simulink model "simulation_car"  (R2020b)
settings: Solver=VariableStepAuto  StartTime=0.0  StopTime=5  RelTol=1e-3
values from neighbouring files (symbols this model uses):
  InitialPosition = zeros(3,1)    [InitSimulink.m]
  InitialVelocity = zeros(3,1)    [InitSimulink.m]
undefined symbols (not defined in the file or in its folder): param
libraries: aerolibutil x10, sharedtransform x6, vrlib x2
settings Model: Creator=rt-2pm2  LastModifiedBy=rt-2pm2

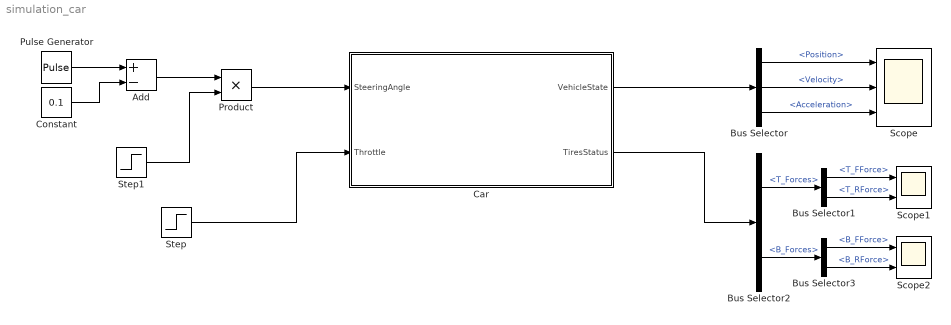
== system simulation_car ==
  Add : Sum  Inputs=+-
  Bus Selector : BusSelector  OutputSignals=StateTranslational.Position,StateTranslational.Velocity,StateTranslational.Acceleration
  Bus Selector1 : BusSelector  OutputSignals=T_FForce,T_RForce
  Bus Selector2 : BusSelector  OutputSignals=T_Forces,B_Forces
  Bus Selector3 : BusSelector  OutputSignals=B_FForce,B_RForce
  Car : Subsystem
  Constant : Constant  Value=0.1
  Product : Product
  Pulse Generator : DiscretePulseGenerator  PulseType=Time based  Amplitude=0.2  Period=10  PulseWidth=5
  Scope : Scope  NumInputPorts=3
  Scope1 : Scope  NumInputPorts=2
  Scope2 : Scope  NumInputPorts=2
  Step : Step  Time=3  Before=3  After=0  SampleTime=0
  Step1 : Step  Time=2  SampleTime=0
  wires:
  Pulse Generator/1 -> Add/1
  Step/1 -> Car/2(Throttle)
  Car/1(VehicleState) -> Bus Selector/1
  Bus Selector/1 -> Scope/1  "<Position>"
  Bus Selector/2 -> Scope/2  "<Velocity>"
  Bus Selector/3 -> Scope/3  "<Acceleration>"
  Car/2(TiresStatus) -> Bus Selector2/1
  Bus Selector1/1 -> Scope1/1  "<T_FForce>"
  Bus Selector1/2 -> Scope1/2  "<T_RForce>"
  Bus Selector2/1 -> Bus Selector1/1  "<T_Forces>"
  Bus Selector3/2 -> Scope2/2  "<B_RForce>"
  Bus Selector3/1 -> Scope2/1  "<B_FForce>"
  Bus Selector2/2 -> Bus Selector3/1  "<B_Forces>"
  Add/1 -> Product/1
  Constant/1 -> Add/2
  Product/1 -> Car/1(SteeringAngle)
  Step1/1 -> Product/2

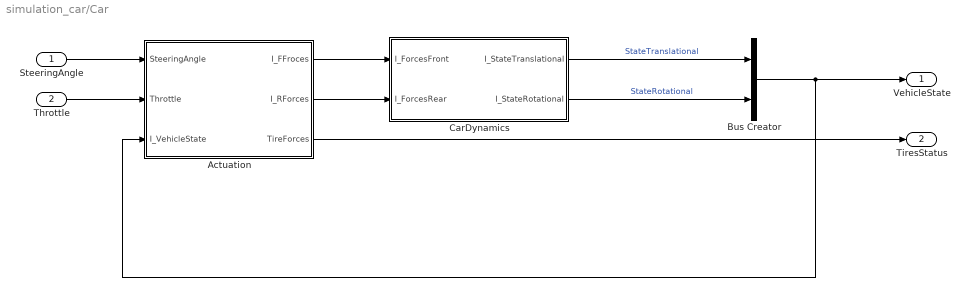
== system simulation_car/Car ==
  SteeringAngle : Inport
  Throttle : Inport  Port=2
  Actuation : Subsystem
  Bus Creator : BusCreator  Inputs=2
  CarDynamics : Subsystem  mask{CarMass=param.m, FrontArmLength=param.a, RearArmLength=param.b, MomentOfInertia=param.Iz}
      mask prompts: CarMass "Car Mass"; FrontArmLength "Front Arm Length"; RearArmLength "Rear Arm Length"; MomentOfInertia "Rotational Inertia"
  VehicleState : Outport
  TiresStatus : Outport  Port=2
  wires:
  CarDynamics/2(I_StateRotational) -> Bus Creator/2  "StateRotational"
  SteeringAngle/1 -> Actuation/1(SteeringAngle)
  CarDynamics/1(I_StateTranslational) -> Bus Creator/1  "StateTranslational"
  Bus Creator/1 -> VehicleState/1, Actuation/3(I_VehicleState)
  Actuation/1(I_FFroces) -> CarDynamics/1(I_ForcesFront)
  Throttle/1 -> Actuation/2(Throttle)
  Actuation/2(I_RForces) -> CarDynamics/2(I_ForcesRear)
  Actuation/3(TireForces) -> TiresStatus/1

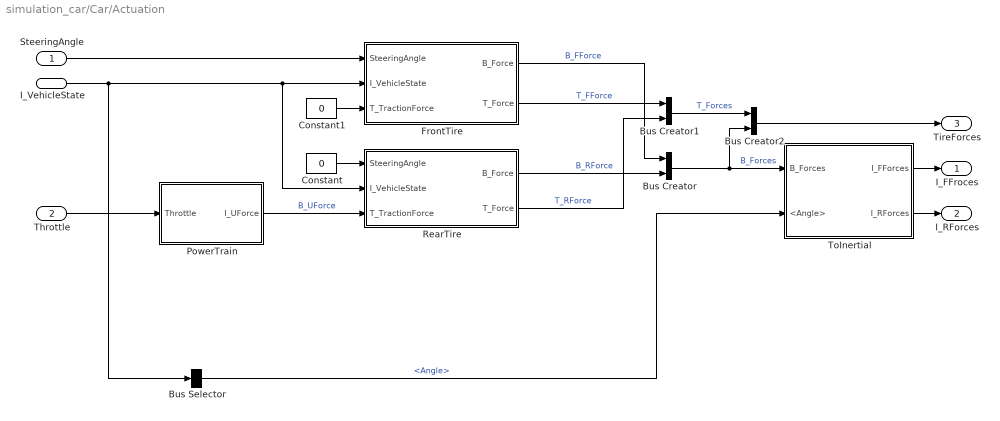
== system simulation_car/Car/Actuation ==
  SteeringAngle : Inport
  Throttle : Inport  Port=2
  I_VehicleState : Inport  Port=3
  Bus Creator : BusCreator  Inputs=2
  Bus Creator1 : BusCreator  Inputs=2
  Bus Creator2 : BusCreator  Inputs=2
  Bus Selector : BusSelector  OutputSignals=StateRotational.Angle
  Constant : Constant  Value=0
  Constant1 : Constant  Value=0
  FrontTire : Subsystem  mask{Arm=[param.a; 0; 0], TireCoeff=param.C_af}
      mask prompts: Arm "Wheel Displacement"; TireCoeff "Tire Coefficient"
      mask Display: image('/home/rt-2pm2/Documents/MATLAB/CIS/lanekeeping_supervision/Simulink/images/tire2.png'); % Use "Edit Image" on toolstrip to change.
  PowerTrain : Subsystem
  RearTire : Subsystem  mask{Arm=[param.a; 0; 0], TireCoeff=param.C_af}
      mask prompts: Arm "Wheel Displacement"; TireCoeff "Tire Coefficient"
      mask Display: image('/home/rt-2pm2/Documents/MATLAB/CIS/lanekeeping_supervision/Simulink/images/tire2.png'); % Use "Edit Image" on toolstrip to change.
  ToInertial : Subsystem
  I_FFroces : Outport
  I_RForces : Outport  Port=2
  TireForces : Outport  Port=3
  wires:
  PowerTrain/1(I_UForce) -> RearTire/3(T_TractionForce)  "B_UForce"
  SteeringAngle/1 -> FrontTire/1(SteeringAngle)
  Throttle/1 -> PowerTrain/1(Throttle)
  I_VehicleState/1 -> Bus Selector/1, RearTire/2(I_VehicleState), FrontTire/2(I_VehicleState)
  Constant/1 -> RearTire/1(SteeringAngle)
  FrontTire/1(B_Force) -> Bus Creator/1  "B_FForce"
  RearTire/1(B_Force) -> Bus Creator/2  "B_RForce"
  Bus Selector/1 -> ToInertial/2(<Angle>)  "<Angle>"
  ToInertial/2(I_RForces) -> I_RForces/1
  ToInertial/1(I_FForces) -> I_FFroces/1
  Constant1/1 -> FrontTire/3(T_TractionForce)
  Bus Creator/1 -> Bus Creator2/2, ToInertial/1(B_Forces)  "B_Forces"
  FrontTire/2(T_Force) -> Bus Creator1/1  "T_FForce"
  RearTire/2(T_Force) -> Bus Creator1/2  "T_RForce"
  Bus Creator1/1 -> Bus Creator2/1  "T_Forces"
  Bus Creator2/1 -> TireForces/1

== system simulation_car/Car/CarDynamics ==
  I_ForcesFront : Inport
  I_ForcesRear : Inport  Port=2
  Subsystem : Subsystem
  Subsystem1 : Subsystem
  I_StateTranslational : Outport
  I_StateRotational : Outport  Port=2
  wires:
  Subsystem/1(StateRotational) -> I_StateRotational/1
  I_ForcesFront/1 -> Subsystem/1(FrontForce), Subsystem1/1(FrontForce)
  I_ForcesRear/1 -> Subsystem/2(RearForce), Subsystem1/2(RearForce)
  Subsystem1/1(StateTranslational) -> I_StateTranslational/1

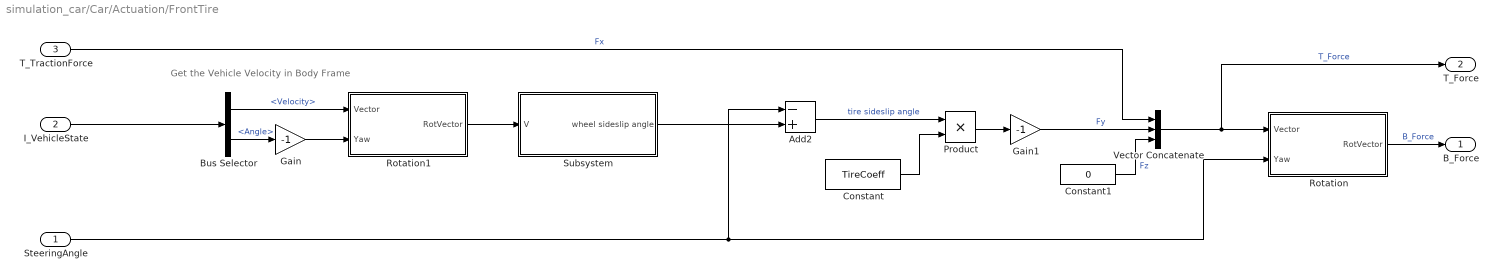
== system simulation_car/Car/Actuation/FrontTire ==
  note: Get the Vehicle Velocity in Body Frame
  SteeringAngle : Inport
  I_VehicleState : Inport  Port=2
  T_TractionForce : Inport  Port=3
  Add2 : Sum  Inputs=-+
  Bus Selector : BusSelector  OutputSignals=StateTranslational.Velocity,StateRotational.Angle
  Constant : Constant  Value=TireCoeff
  Constant1 : Constant  Value=0
  Gain : Gain  Gain=-1
  Gain1 : Gain  Gain=-1
  Product : Product
  Rotation : Subsystem
  Rotation1 : Subsystem
  Subsystem : Subsystem
  Vector Concatenate : Concatenate  NumInputs=3
  B_Force : Outport
  T_Force : Outport  Port=2
  wires:
  Vector Concatenate/1 -> T_Force/1, Rotation/1(Vector)  "T_Force"
  Gain1/1 -> Vector Concatenate/2  "Fy"
  Product/1 -> Gain1/1
  Constant/1 -> Product/2
  Bus Selector/1 -> Rotation1/1(Vector)  "<Velocity>"
  Gain/1 -> Rotation1/2(Yaw)
  Bus Selector/2 -> Gain/1  "<Angle>"
  I_VehicleState/1 -> Bus Selector/1
  Add2/1 -> Product/1  "tire sideslip angle"
  T_TractionForce/1 -> Vector Concatenate/1  "Fx"
  SteeringAngle/1 -> Rotation/2(Yaw), Add2/1
  Rotation/1(RotVector) -> B_Force/1  "B_Force"
  Constant1/1 -> Vector Concatenate/3  "Fz"
  Rotation1/1(RotVector) -> Subsystem/1(V)
  Subsystem/1(wheel sideslip angle) -> Add2/2

== system simulation_car/Car/Actuation/PowerTrain ==
  Throttle : Inport
  Throttle2Force : Gain
  I_UForce : Outport
  wires:
  Throttle/1 -> Throttle2Force/1
  Throttle2Force/1 -> I_UForce/1

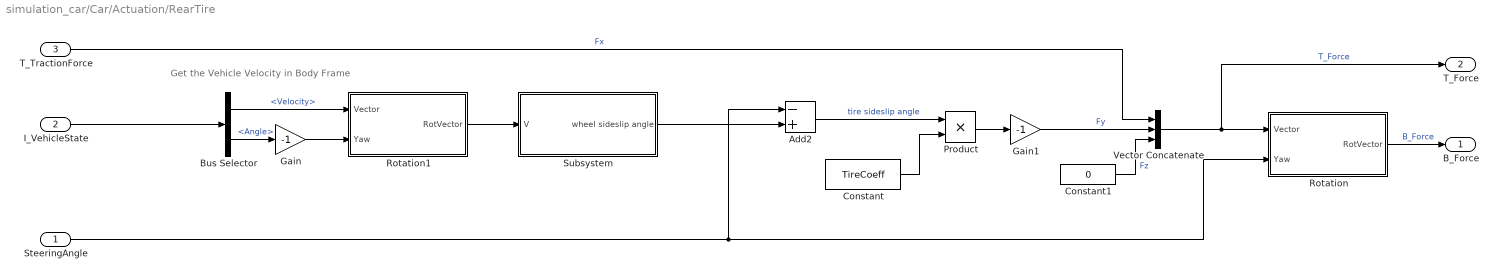
== system simulation_car/Car/Actuation/RearTire ==
  note: Get the Vehicle Velocity in Body Frame
  SteeringAngle : Inport
  I_VehicleState : Inport  Port=2
  T_TractionForce : Inport  Port=3
  Add2 : Sum  Inputs=-+
  Bus Selector : BusSelector  OutputSignals=StateTranslational.Velocity,StateRotational.Angle
  Constant : Constant  Value=TireCoeff
  Constant1 : Constant  Value=0
  Gain : Gain  Gain=-1
  Gain1 : Gain  Gain=-1
  Product : Product
  Rotation : Subsystem
  Rotation1 : Subsystem
  Subsystem : Subsystem
  Vector Concatenate : Concatenate  NumInputs=3
  B_Force : Outport
  T_Force : Outport  Port=2
  wires:
  Subsystem/1(wheel sideslip angle) -> Add2/2
  Rotation1/1(RotVector) -> Subsystem/1(V)
  Constant1/1 -> Vector Concatenate/3  "Fz"
  Rotation/1(RotVector) -> B_Force/1  "B_Force"
  SteeringAngle/1 -> Add2/1, Rotation/2(Yaw)
  T_TractionForce/1 -> Vector Concatenate/1  "Fx"
  Add2/1 -> Product/1  "tire sideslip angle"
  I_VehicleState/1 -> Bus Selector/1
  Bus Selector/2 -> Gain/1  "<Angle>"
  Gain/1 -> Rotation1/2(Yaw)
  Bus Selector/1 -> Rotation1/1(Vector)  "<Velocity>"
  Constant/1 -> Product/2
  Product/1 -> Gain1/1
  Gain1/1 -> Vector Concatenate/2  "Fy"
  Vector Concatenate/1 -> Rotation/1(Vector), T_Force/1  "T_Force"

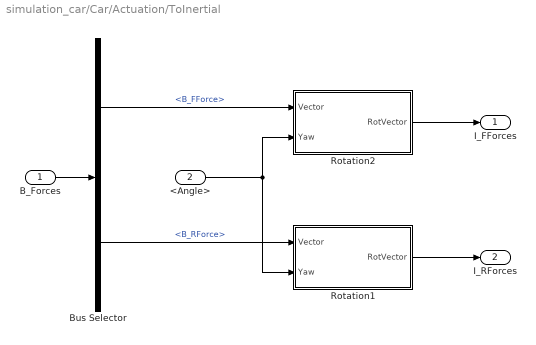
== system simulation_car/Car/Actuation/ToInertial ==
  B_Forces : Inport
  <Angle> : Inport  Port=2
  Bus Selector : BusSelector  OutputSignals=B_FForce,B_RForce
  Rotation1 : Subsystem
  Rotation2 : Subsystem
  I_FForces : Outport
  I_RForces : Outport  Port=2
  wires:
  <Angle>/1 -> Rotation1/2(Yaw), Rotation2/2(Yaw)
  B_Forces/1 -> Bus Selector/1
  Rotation1/1(RotVector) -> I_RForces/1
  Bus Selector/1 -> Rotation2/1(Vector)  "<B_FForce>"
  Rotation2/1(RotVector) -> I_FForces/1
  Bus Selector/2 -> Rotation1/1(Vector)  "<B_RForce>"

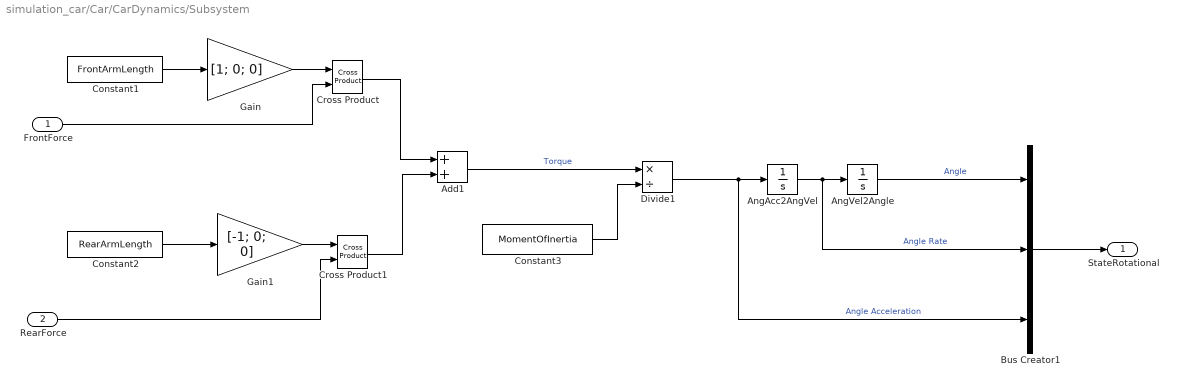
== system simulation_car/Car/CarDynamics/Subsystem ==
  FrontForce : Inport
  RearForce : Inport  Port=2
  Add1 : Sum
  AngAcc2AngVel : Integrator
  AngVel2Angle : Integrator
  Bus Creator1 : BusCreator  Inputs=3
  Constant1 : Constant  Value=FrontArmLength
  Constant2 : Constant  Value=RearArmLength
  Constant3 : Constant  Value=MomentOfInertia
  Cross Product : vrlib/Utilities/Cross Product
  Cross Product1 : vrlib/Utilities/Cross Product
  Divide1 : Product  Inputs=*/
  Gain : Gain  Gain=[1; 0; 0]
  Gain1 : Gain  Gain=[-1; 0; 0]
  StateRotational : Outport
  wires:
  Gain1/1 -> Cross Product1/1
  Gain/1 -> Cross Product/1
  Constant1/1 -> Gain/1
  Cross Product1/1 -> Add1/2
  AngAcc2AngVel/1 -> Bus Creator1/2, AngVel2Angle/1  "Angle Rate"
  Constant3/1 -> Divide1/2
  Add1/1 -> Divide1/1  "Torque"
  AngVel2Angle/1 -> Bus Creator1/1  "Angle"
  RearForce/1 -> Cross Product1/2
  Divide1/1 -> Bus Creator1/3, AngAcc2AngVel/1  "Angle Acceleration"
  Cross Product/1 -> Add1/1
  Constant2/1 -> Gain1/1
  Bus Creator1/1 -> StateRotational/1
  FrontForce/1 -> Cross Product/2

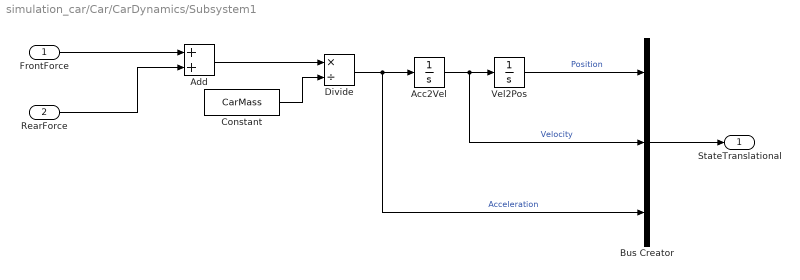
== system simulation_car/Car/CarDynamics/Subsystem1 ==
  FrontForce : Inport
  RearForce : Inport  Port=2
  Acc2Vel : Integrator  InitialCondition=InitialVelocity
  Add : Sum
  Bus Creator : BusCreator  Inputs=3
  Constant : Constant  Value=CarMass
  Divide : Product  Inputs=*/
  Vel2Pos : Integrator  InitialCondition=InitialPosition
  StateTranslational : Outport
  wires:
  Constant/1 -> Divide/2
  FrontForce/1 -> Add/1
  Bus Creator/1 -> StateTranslational/1
  RearForce/1 -> Add/2
  Add/1 -> Divide/1
  Acc2Vel/1 -> Bus Creator/2, Vel2Pos/1  "Velocity"
  Vel2Pos/1 -> Bus Creator/1  "Position"
  Divide/1 -> Bus Creator/3, Acc2Vel/1  "Acceleration"

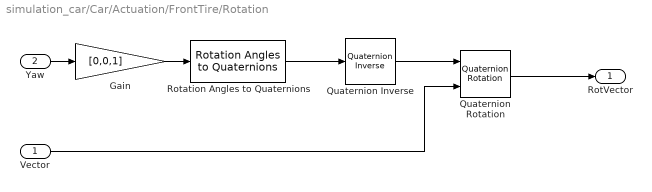
== system simulation_car/Car/Actuation/FrontTire/Rotation ==
  Vector : Inport
  Yaw : Inport  Port=2
  Gain : Gain  Gain=[0,0,1]
  Quaternion Inverse : aerolibutil/Quaternion Inverse
  Quaternion Rotation : aerolibutil/Quaternion Rotation
  Rotation Angles to Quaternions : sharedtransform/Rotation Angles to Quaternions  rotationOrder=XYZ  aMode=aMode
      settings: SourceProductBaseCode=AE,PW,MT,UV,VE,VP
  RotVector : Outport
  wires:
  Rotation Angles to Quaternions/1 -> Quaternion Inverse/1
  Gain/1 -> Rotation Angles to Quaternions/1
  Yaw/1 -> Gain/1
  Quaternion Rotation/1 -> RotVector/1
  Vector/1 -> Quaternion Rotation/2
  Quaternion Inverse/1 -> Quaternion Rotation/1

== system simulation_car/Car/Actuation/FrontTire/Rotation1 ==
  Vector : Inport
  Yaw : Inport  Port=2
  Gain : Gain  Gain=[0,0,1]
  Quaternion Rotation : aerolibutil/Quaternion Rotation
  Rotation Angles to Quaternions : sharedtransform/Rotation Angles to Quaternions  rotationOrder=ZYX  aMode=aMode
      settings: SourceProductBaseCode=AE,PW,MT,UV,VE,VP
  RotVector : Outport
  wires:
  Vector/1 -> Quaternion Rotation/2
  Quaternion Rotation/1 -> RotVector/1
  Yaw/1 -> Gain/1
  Gain/1 -> Rotation Angles to Quaternions/1
  Rotation Angles to Quaternions/1 -> Quaternion Rotation/1

== system simulation_car/Car/Actuation/FrontTire/Subsystem ==
  V : Inport
  MATLAB Function : MATLAB Function  TreatAsAtomicUnit=on
  wheel sideslip angle : Outport
  wires:
  MATLAB Function/1(beta) -> wheel sideslip angle/1  "wheel sideslip angle"
  V/1 -> MATLAB Function/1(V)

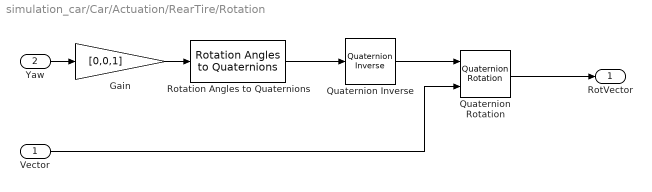
== system simulation_car/Car/Actuation/RearTire/Rotation ==
  Vector : Inport
  Yaw : Inport  Port=2
  Gain : Gain  Gain=[0,0,1]
  Quaternion Inverse : aerolibutil/Quaternion Inverse
  Quaternion Rotation : aerolibutil/Quaternion Rotation
  Rotation Angles to Quaternions : sharedtransform/Rotation Angles to Quaternions  rotationOrder=XYZ  aMode=aMode
      settings: SourceProductBaseCode=AE,PW,MT,UV,VE,VP
  RotVector : Outport
  wires:
  Quaternion Inverse/1 -> Quaternion Rotation/1
  Vector/1 -> Quaternion Rotation/2
  Quaternion Rotation/1 -> RotVector/1
  Yaw/1 -> Gain/1
  Gain/1 -> Rotation Angles to Quaternions/1
  Rotation Angles to Quaternions/1 -> Quaternion Inverse/1

== system simulation_car/Car/Actuation/RearTire/Rotation1 ==
  Vector : Inport
  Yaw : Inport  Port=2
  Gain : Gain  Gain=[0,0,1]
  Quaternion Rotation : aerolibutil/Quaternion Rotation
  Rotation Angles to Quaternions : sharedtransform/Rotation Angles to Quaternions  rotationOrder=ZYX  aMode=aMode
      settings: SourceProductBaseCode=AE,PW,MT,UV,VE,VP
  RotVector : Outport
  wires:
  Rotation Angles to Quaternions/1 -> Quaternion Rotation/1
  Gain/1 -> Rotation Angles to Quaternions/1
  Yaw/1 -> Gain/1
  Quaternion Rotation/1 -> RotVector/1
  Vector/1 -> Quaternion Rotation/2

== system simulation_car/Car/Actuation/RearTire/Subsystem ==
  V : Inport
  MATLAB Function : MATLAB Function  TreatAsAtomicUnit=on
  wheel sideslip angle : Outport
  wires:
  V/1 -> MATLAB Function/1(V)
  MATLAB Function/1(beta) -> wheel sideslip angle/1  "wheel sideslip angle"

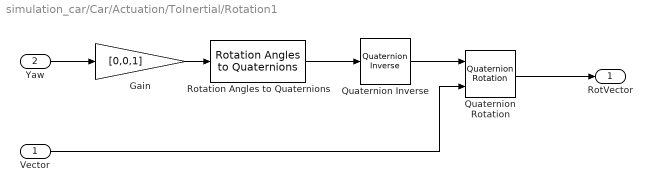
== system simulation_car/Car/Actuation/ToInertial/Rotation1 ==
  Vector : Inport
  Yaw : Inport  Port=2
  Gain : Gain  Gain=[0,0,1]
  Quaternion Inverse : aerolibutil/Quaternion Inverse
  Quaternion Rotation : aerolibutil/Quaternion Rotation
  Rotation Angles to Quaternions : sharedtransform/Rotation Angles to Quaternions  rotationOrder=XYZ  aMode=aMode
      settings: SourceProductBaseCode=AE,PW,MT,UV,VE,VP
  RotVector : Outport
  wires:
  Quaternion Inverse/1 -> Quaternion Rotation/1
  Vector/1 -> Quaternion Rotation/2
  Quaternion Rotation/1 -> RotVector/1
  Yaw/1 -> Gain/1
  Gain/1 -> Rotation Angles to Quaternions/1
  Rotation Angles to Quaternions/1 -> Quaternion Inverse/1

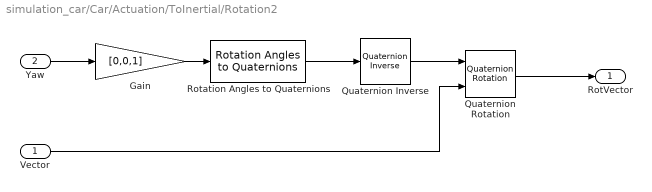
== system simulation_car/Car/Actuation/ToInertial/Rotation2 ==
  Vector : Inport
  Yaw : Inport  Port=2
  Gain : Gain  Gain=[0,0,1]
  Quaternion Inverse : aerolibutil/Quaternion Inverse
  Quaternion Rotation : aerolibutil/Quaternion Rotation
  Rotation Angles to Quaternions : sharedtransform/Rotation Angles to Quaternions  rotationOrder=XYZ  aMode=aMode
      settings: SourceProductBaseCode=AE,PW,MT,UV,VE,VP
  RotVector : Outport
  wires:
  Rotation Angles to Quaternions/1 -> Quaternion Inverse/1
  Gain/1 -> Rotation Angles to Quaternions/1
  Yaw/1 -> Gain/1
  Quaternion Rotation/1 -> RotVector/1
  Vector/1 -> Quaternion Rotation/2
  Quaternion Inverse/1 -> Quaternion Rotation/1

== matlab function simulation_car/Car/Actuation/FrontTire/Subsystem/MATLAB Function ==
  data: V input; beta output
function beta = ComputeWheelSideslipAngle(V)
% Compute the Wheel Sideslip Angle
beta = 0;

Vx = V(1);
Vy = V(2);

if (Vx > 0.001)
    beta = atan(Vy / Vx);
end

end

== matlab function simulation_car/Car/Actuation/RearTire/Subsystem/MATLAB Function ==
  data: V input; beta output
function beta = ComputeWheelSideslipAngle(V)
% Compute the Wheel Sideslip Angle
beta = 0;

Vx = V(1);
Vy = V(2);

if (Vx > 0.001)
    beta = atan(Vy / Vx);
end

end
